simulink model "NominalEncounter"  (R2021b)
settings: Solver=ode45  StartTime=0.0  StopTime=90  RelTol=1e-3  EnableMultiTasking=on
undefined symbols (not defined in the file or in its folder): radarParamConverter, Subsystem
libraries: Tracked_Radar_Block x3, NominalTrajectory x2, BasicAircraftDynamicsBlock x2, GPS_INS_Block x2, CommonMetricsBlock x1, SLoWCBlock x1, WellClearMetricsBlock x1, StopConditionsBlock x1, aerolibutil x1, sph2cart x1
settings Model: Creator=JO20596  LastModifiedBy=lydiazeleke
settings SolverCC: AlgebraicLoopSolver=TrustRegion
settings DataIOCC: LimitDataPoints=on  MaxDataPoints=10000  SignalLoggingSaveFormat=ModelDataLogs  SaveState=on  ReturnWorkspaceOutputs=off  StateSaveName=xoutNew  OutputSaveName=youtNew
settings OptimizationCC: ExpressionDepthLimit=2147483647  LifeSpan=inf
settings DebuggingCC: UnderspecifiedInitializationDetection=Classic  MergeDetectMultiDrivingBlocksExec=none  SolverPrmCheckMsg=warning  FcnCallInpInsideContextMsg=warning  StateNameClashWarn=warning  SFUnexpectedBacktrackingDiag=warning  SFNoUnconditionalDefaultTransitionDiag=warning  SFExecutionAtInitializationDiag=none  SFMachineParentedDataDiag=warning  ArithmeticOperatorsInVariantConditions=warning
settings HardwareCC: ProdBitPerPointer=32  ProdBitPerSizeT=32  ProdBitPerPtrDiffT=32  ProdLargestAtomicFloat=None  ProdIntDivRoundTo=Undefined  ProdEndianess=Unspecified  ProdWordSize=32  ProdHWDeviceType=32-bit Generic
settings ModelReferenceCC: PropagateSignalLabelsOutOfModel=off
settings SFSimCC: SimUseLocalCustomCode=off  CustomCodeUndefinedFunction=UseInterfaceOnly
settings RTWCC: RTWUseLocalCustomCode=off
settings CodeAppCC: StateflowObjectComments=on
settings GRTTargetCC: TargetLangStandard=C89/C90 (ANSI)  CombineOutputUpdateFcns=off  GRTInterface=on
settings ConfigComp: CovMetricSettings=dw  CovSaveCumulativeToWorkspaceVar=on  CovSaveSingleToWorkspaceVar=on  CovExternalEMLEnable=off

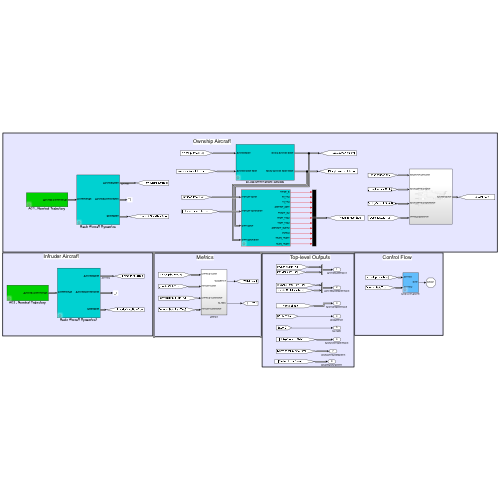
[thumbnail: Simulink's stored preview of the top-level diagram]
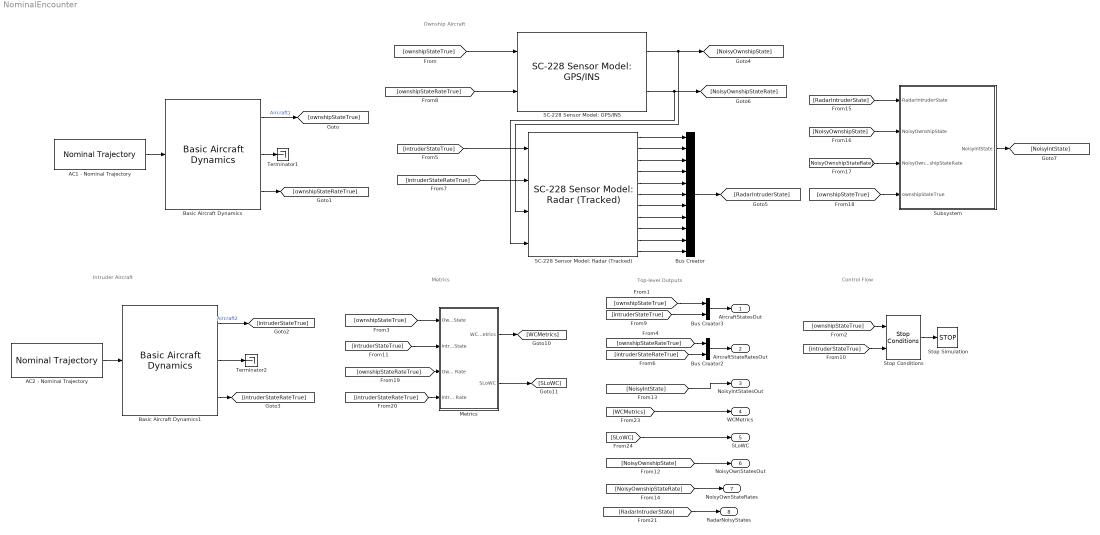
== system NominalEncounter ==
  note: Metrics
  note: Control Flow
  note: Top-level Outputs
  note: Ownship Aircraft
  note: Intruder Aircraft
  AC1 - Nominal Trajectory : NominalTrajectory/Nominal Trajectory  eventFilename=event1.mat  ts=.1
  AC2 - Nominal Trajectory : NominalTrajectory/Nominal Trajectory  eventFilename=event2.mat  ts=.1
  Basic Aircraft Dynamics : BasicAircraftDynamicsBlock/Basic Aircraft Dynamics  ts_dynamics=.1  v_ftps_0=ac1dyn_v_ftps  N_ft_0=ac1dyn_N_ft  E_ft_0=ac1dyn_E_ft  h_ft_0=ac1dyn_h_ft  psi_rad_0=ac1dyn_psi_rad  theta_rad_0=ac1dyn_theta_rad  phi_rad_0=ac1dyn_phi_rad  a_ftpss_0=ac1dyn_a_ftpss  v_ftps_max=ac1dyn_con.maxAirspeed_ftps  v_ftps_min=ac1dyn_con.minAirspeed_ftps  dv_ftpss_max=ac1dyn_con.maxAcceleration_ftpss  dv_ftpss_min=ac1dyn_con.minAcceleration_ftpss  dh_ftps_max=ac1dyn_con.maxVerticalRate_ftps  dh_ftps_min=ac1dyn_con.minVerticalRate_ftps  q_radps_max=ac1dyn_con.maxPitchRate_radps  phi_rad_max=ac1dyn_con.maxBankAngle_rad  dphi_radps_max=ac1dyn_con.maxRollRate_radps  r_radps_max=ac1dyn_con.maxYawRate_radps  pNUM=ac1dyn_con.dynamicsNumeratorRollRate  pDEN=ac1dyn_con.dynamicsDenominatorRollRate  hNUM=ac1dyn_con.dynamicsNumeratorVerticalRate  hDEN=ac1dyn_con.dynamicsDenominatorVerticalRate  rNUM=ac1dyn_con.dynamicsNumeratorYawRate  rDEN=ac1dyn_con.dynamicsDenominatorYawRate  lat0_rad=ac1dyn_lat0_rad  lon0_rad=ac1dyn_lon0_rad  alt_ft=ac1dyn_alt0_ft
  Basic Aircraft Dynamics1 : BasicAircraftDynamicsBlock/Basic Aircraft Dynamics  ts_dynamics=.1  v_ftps_0=ac2dyn_v_ftps  N_ft_0=ac2dyn_N_ft  E_ft_0=ac2dyn_E_ft  h_ft_0=ac2dyn_h_ft  psi_rad_0=ac2dyn_psi_rad  theta_rad_0=ac2dyn_theta_rad  phi_rad_0=ac2dyn_phi_rad  a_ftpss_0=ac2dyn_a_ftpss  v_ftps_max=ac2dyn_con.maxAirspeed_ftps  v_ftps_min=ac2dyn_con.minAirspeed_ftps  dv_ftpss_max=ac2dyn_con.maxAcceleration_ftpss  dv_ftpss_min=ac2dyn_con.minAcceleration_ftpss  dh_ftps_max=ac2dyn_con.maxVerticalRate_ftps  dh_ftps_min=ac2dyn_con.minVerticalRate_ftps  q_radps_max=ac2dyn_con.maxPitchRate_radps  phi_rad_max=ac2dyn_con.maxBankAngle_rad  dphi_radps_max=ac2dyn_con.maxRollRate_radps  r_radps_max=ac2dyn_con.maxYawRate_radps  pNUM=ac2dyn_con.dynamicsNumeratorRollRate  pDEN=ac2dyn_con.dynamicsDenominatorRollRate  hNUM=ac2dyn_con.dynamicsNumeratorVerticalRate  hDEN=ac2dyn_con.dynamicsDenominatorVerticalRate  rNUM=ac2dyn_con.dynamicsNumeratorYawRate  rDEN=ac2dyn_con.dynamicsDenominatorYawRate  lat0_rad=ac2dyn_lat0_rad  lon0_rad=ac2dyn_lon0_rad  alt_ft=ac2dyn_alt0_ft
  Bus Creator : BusCreator  Inputs=11
  Bus Creator2 : BusCreator  Inputs=2
  Bus Creator3 : BusCreator  Inputs=2
  Metrics : Subsystem
  SC-228 Sensor Model: GPS/INS : GPS_INS_Block/SC-228 Sensor Model: GPS//INS  dt_s=uas_own_dt_s  perfect=uas_own_usePerfectAlt  lat0_rad=ac1dyn_lat0_rad  lon0_rad=ac1dyn_lon0_rad  alt0_ft=ac1dyn_alt0_ft  vx_random_stddev_ftps=uas_own_vy_random_stddev_ftps  vx_bias_ftps=uas_own_vy_bias_ftps  vx_tau_s=uas_own_vy_tau_s  seed4=uas_own_seed4  vy_random_stddev_ftps=uas_own_vx_random_stddev_ftps  vy_bias_ftps=uas_own_vx_bias_ftps  vy_tau_s=uas_own_vx_tau_s  seed5=uas_own_seed5  psi_random_stddev_rad=uas_own_psi_random_stddev_rad  seed1=uas_own_seed1  phi_random_stddev_rad=uas_own_phi_random_stddev_rad  seed2=uas_own_seed2  theta_random_stddev_rad=uas_own_theta_random_stddev_rad  seed3=uas_own_seed3  seed6=uas_own_seed6  y_random_stddev_ft=uas_own_y_random_stddev_ft  y_bias_ft=uas_own_y_bias_ft  y_tau_s=uas_own_y_tau_s  seed7=uas_own_seed7  x_random_stddev_ft=uas_own_x_random_stddev_ft  x_bias_ft=uas_own_x_bias_ft  x_tau_s=uas_own_x_tau_s  seed8=uas_own_seed8  seed9=uas_own_seed9  seed10=uas_own_seed10  altQuant_ft=uas_own_altQuant_ft
  SC-228 Sensor Model: Radar (Tracked) : Tracked_Radar_Block/SC-228 Sensor Model: Radar (Tracked)  dt_s=uas_rdr_trckd_dt_s  lat0_rad=ac1dyn_lat0_rad  lon0_rad=ac1dyn_lon0_rad  alt0_ft=ac1dyn_alt0_ft  sns_for_azimuth_deg=uas_rdr_trckd_sns_for_azimuth_deg  sns_for_elevation_deg=uas_rdr_trckd_sns_for_elevation_deg  debugMode=uas_rdr_trckd_debugMode  rng_random_stddev_ft=uas_rdr_trckd_rng_random_stddev_ft  rng_bias_ft=uas_rdr_trckd_rng_bias_ft  rng_tau_s=uas_rdr_trckd_rng_tau_s  seed1=uas_rdr_trckd_seed1  RCPR_Mode=uas_rdr_trckd_RCPR_Mode  RCPR_Range_ft=uas_rdr_trckd_RCPR_Range_ft  az_random_stddev_rad=uas_rdr_trckd_az_random_stddev_rad  az_bias_rad=uas_rdr_trckd_az_bias_rad  az_tau_s=uas_rdr_trckd_az_tau_s  seed2=uas_rdr_trckd_seed2  el_random_stddev_rad=uas_rdr_trckd_el_random_stddev_rad  el_bias_rad=uas_rdr_trckd_el_bias_rad  el_tau_s=uas_rdr_trckd_el_tau_s  seed3=uas_rdr_trckd_seed3  rngdot_random_stddev_ftps=uas_rdr_trckd_rngdot_random_stddev_ftps  rngdot_bias_ftps=uas_rdr_trckd_rngdot_bias_ftps  rngdot_tau_s=uas_rdr_trckd_rngdot_tau_s  seed4=uas_rdr_trckd_seed4  covRAE=uas_rdr_trckd_reported_errorCovRAE
  Stop Conditions : StopConditionsBlock/Stop Conditions  range_limit_ft=stop_range_ft  altitude_limit_ft=stop_altitude_ft
  Stop Simulation : Stop
  Subsystem : Subsystem  AncestorBlock=radarParamConverter/Subsystem
  Terminator1 : Terminator
  Terminator2 : Terminator
  AircraftStatesOut : Outport  VectorParamsAs1DForOutWhenUnconnected=off
  AircraftStateRatesOut : Outport  Port=2  VectorParamsAs1DForOutWhenUnconnected=off
  NoisyIntStatesOut : Outport  Port=3  VectorParamsAs1DForOutWhenUnconnected=off
  WCMetrics : Outport  Port=4  VectorParamsAs1DForOutWhenUnconnected=off
  SLoWC : Outport  Port=5  VectorParamsAs1DForOutWhenUnconnected=off
  NoisyOwnStatesOut : Outport  Port=6  VectorParamsAs1DForOutWhenUnconnected=off
  NoisyOwnStateRates : Outport  Port=7  VectorParamsAs1DForOutWhenUnconnected=off
  RadarNoisyStates : Outport  Port=8  VectorParamsAs1DForOutWhenUnconnected=off
  wires:
  Bus Creator2/1 -> AircraftStateRatesOut/1
  Stop Conditions/1 -> Stop Simulation/1
  [ownshipStateTrue] -> Stop Conditions/1
  [ownshipStateRateTrue] -> Bus Creator2/1
  [intruderStateRateTrue] -> Bus Creator2/2
  [intruderStateTrue] -> Stop Conditions/2
  [ownshipStateTrue] -> Metrics/1(Ownship State)
  [intruderStateTrue] -> Metrics/2(Intruder State)
  [ownshipStateRateTrue] -> Metrics/3(Ownship State Rate)
  [intruderStateRateTrue] -> Metrics/4(Intruder State Rate)
  Metrics/1(WCMetrics) -> [WCMetrics]
  Metrics/2(SLoWC) -> [SLoWC]
  [WCMetrics] -> WCMetrics/1
  [SLoWC] -> SLoWC/1
  Basic Aircraft Dynamics1/3 -> [intruderStateRateTrue]
  Basic Aircraft Dynamics/2 -> Terminator1/1
  AC1 - Nominal Trajectory/1 -> Basic Aircraft Dynamics/1
  Basic Aircraft Dynamics1/1 -> [intruderStateTrue]  "Aircraft2"
  Basic Aircraft Dynamics1/2 -> Terminator2/1
  AC2 - Nominal Trajectory/1 -> Basic Aircraft Dynamics1/1
  Basic Aircraft Dynamics/1 -> [ownshipStateTrue]  "Aircraft1"
  Basic Aircraft Dynamics/3 -> [ownshipStateRateTrue]
  [intruderStateTrue] -> SC-228 Sensor Model: Radar (Tracked)/1
  [NoisyIntState] -> NoisyIntStatesOut/1
  [ownshipStateTrue] -> Bus Creator3/1
  [intruderStateTrue] -> Bus Creator3/2
  Bus Creator3/1 -> AircraftStatesOut/1
  SC-228 Sensor Model: GPS/INS/1 -> SC-228 Sensor Model: Radar (Tracked)/3, [NoisyOwnshipState]
  SC-228 Sensor Model: GPS/INS/2 -> SC-228 Sensor Model: Radar (Tracked)/4, [NoisyOwnshipStateRate]
  [ownshipStateTrue] -> SC-228 Sensor Model: GPS/INS/1
  [ownshipStateRateTrue] -> SC-228 Sensor Model: GPS/INS/2
  [intruderStateRateTrue] -> SC-228 Sensor Model: Radar (Tracked)/2
  [NoisyOwnshipStateRate] -> NoisyOwnStateRates/1
  [NoisyOwnshipState] -> NoisyOwnStatesOut/1
  SC-228 Sensor Model: Radar (Tracked)/1 -> Bus Creator/1
  SC-228 Sensor Model: Radar (Tracked)/2 -> Bus Creator/2
  SC-228 Sensor Model: Radar (Tracked)/3 -> Bus Creator/3
  SC-228 Sensor Model: Radar (Tracked)/4 -> Bus Creator/4
  SC-228 Sensor Model: Radar (Tracked)/5 -> Bus Creator/5
  SC-228 Sensor Model: Radar (Tracked)/6 -> Bus Creator/6
  SC-228 Sensor Model: Radar (Tracked)/7 -> Bus Creator/7
  SC-228 Sensor Model: Radar (Tracked)/8 -> Bus Creator/8
  SC-228 Sensor Model: Radar (Tracked)/9 -> Bus Creator/9
  SC-228 Sensor Model: Radar (Tracked)/10 -> Bus Creator/10
  SC-228 Sensor Model: Radar (Tracked)/11 -> Bus Creator/11
  Bus Creator/1 -> [RadarIntruderState]
  [RadarIntruderState] -> Subsystem/1(RadarIntruderState)
  [NoisyOwnshipState] -> Subsystem/2(NoisyOwnshipState)
  [NoisyOwnshipStateRate] -> Subsystem/3(NoisyOwnshipStateRate)
  Subsystem/1(NoisyIntState) -> [NoisyIntState]
  [ownshipStateTrue] -> Subsystem/4(ownshipStateTrue)
  [RadarIntruderState] -> RadarNoisyStates/1

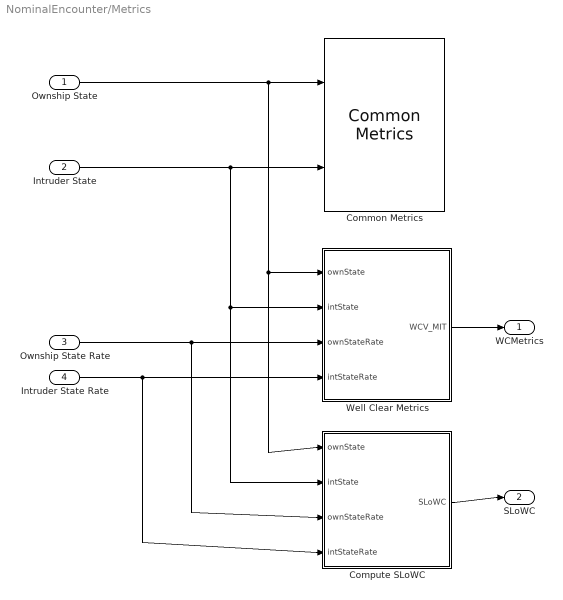
== system NominalEncounter/Metrics ==
  Ownship State : Inport
  Intruder State : Inport  Port=2
  Ownship State Rate : Inport  Port=3
  Intruder State Rate : Inport  Port=4
  Common Metrics : CommonMetricsBlock/Common Metrics
  Compute SLoWC : Subsystem  mask{DMOD=4000, tauMod=35, altDiff=450}
      mask prompts: altDiff "Altitude Difference Threshold:"
  Well Clear Metrics : Subsystem
  WCMetrics : Outport  VectorParamsAs1DForOutWhenUnconnected=off
  SLoWC : Outport  Port=2  VectorParamsAs1DForOutWhenUnconnected=off
  wires:
  Ownship State/1 -> Common Metrics/1, Well Clear Metrics/1(ownState), Compute SLoWC/1(ownState)
  Intruder State/1 -> Common Metrics/2, Well Clear Metrics/2(intState), Compute SLoWC/2(intState)
  Ownship State Rate/1 -> Well Clear Metrics/3(ownStateRate), Compute SLoWC/3(ownStateRate)
  Intruder State Rate/1 -> Well Clear Metrics/4(intStateRate), Compute SLoWC/4(intStateRate)
  Well Clear Metrics/1(WCV_MIT) -> WCMetrics/1
  Compute SLoWC/1(SLoWC) -> SLoWC/1

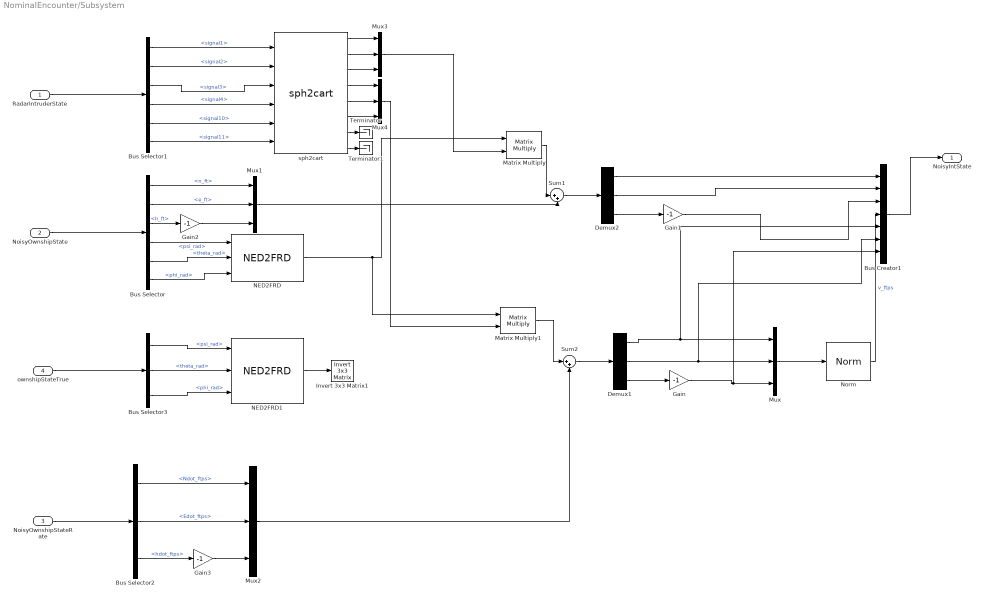
== system NominalEncounter/Subsystem ==
  RadarIntruderState : Inport
  NoisyOwnshipState : Inport  Port=2  OutDataTypeStr=Bus: AircraftState
  NoisyOwnshipStateRate : Inport  Port=3  OutDataTypeStr=Bus: AircraftStateRate
  ownshipStateTrue : Inport  Port=4  OutDataTypeStr=Bus: AircraftState
  Bus Creator1 : BusCreator  Inputs=7
  Bus Selector : BusSelector  OutputSignals=n_ft,e_ft,h_ft,psi_rad,theta_rad,phi_rad
  Bus Selector1 : BusSelector  OutputSignals=signal1,signal2,signal3,signal4,signal10,signal11
  Bus Selector2 : BusSelector  OutputSignals=Ndot_ftps,Edot_ftps,hdot_ftps
  Bus Selector3 : BusSelector  OutputSignals=psi_rad,theta_rad,phi_rad
  Demux1 : Demux  Outputs=3
  Demux2 : Demux  Outputs=3
  Gain{,1..3} (4 alike) : Gain  Gain=-1
  Invert 3x3 Matrix1 : aerolibutil/Invert  3x3 Matrix
  Matrix Multiply : Product  Multiplication=Matrix(*)
  Matrix Multiply1 : Product  Multiplication=Matrix(*)
  Mux{,1..4} (5 alike) : Mux  Inputs=3
  NED2FRD : Tracked_Radar_Block/SC-228 Sensor Model: Radar (Tracked)/NED2FRD  SystemSampleTime=-1  VariantActivationTime=update diagram  Latency=0  AutoFrameSizeCalculation=off
  NED2FRD1 : Tracked_Radar_Block/SC-228 Sensor Model: Radar (Tracked)/NED2FRD  SystemSampleTime=-1  VariantActivationTime=update diagram  Latency=0  AutoFrameSizeCalculation=off
  Norm : GPS_INS_Block/SC-228 Sensor Model: GPS//INS/Norm  SystemSampleTime=-1  VariantActivationTime=update diagram  Latency=0  AutoFrameSizeCalculation=off
  Sum1 : Sum  Inputs=|++
  Sum2 : Sum  Inputs=|++
  Terminator : Terminator
  Terminator1 : Terminator
  sph2cart : sph2cart/sph2cart  SystemSampleTime=-1  VariantActivationTime=update diagram  Latency=0  AutoFrameSizeCalculation=off
      settings: SourceProductName=CASSATTv6: Signals Library
  NoisyIntState : Outport  VectorParamsAs1DForOutWhenUnconnected=off
  wires:
  NoisyOwnshipState/1 -> Bus Selector/1
  RadarIntruderState/1 -> Bus Selector1/1
  NoisyOwnshipStateRate/1 -> Bus Selector2/1
  Bus Selector/4 -> NED2FRD/1  "<psi_rad>"
  Bus Selector/5 -> NED2FRD/2  "<theta_rad>"
  Bus Selector/6 -> NED2FRD/3  "<phi_rad>"
  Bus Selector/1 -> Mux1/1  "<n_ft>"
  Bus Selector/2 -> Mux1/2  "<e_ft>"
  Bus Selector2/1 -> Mux2/1  "<Ndot_ftps>"
  Bus Selector2/2 -> Mux2/2  "<Edot_ftps>"
  Matrix Multiply/1 -> Sum1/1
  Mux1/1 -> Sum1/2
  Sum1/1 -> Demux2/1
  Sum2/1 -> Demux1/1
  Mux2/1 -> Sum2/2
  Matrix Multiply1/1 -> Sum2/1
  Demux2/2 -> Bus Creator1/2
  Demux1/1 -> Bus Creator1/5, Mux/1
  Demux1/2 -> Bus Creator1/6, Mux/2
  Mux/1 -> Norm/1
  Demux1/3 -> Gain/1
  Demux2/3 -> Gain1/1
  Gain1/1 -> Bus Creator1/3
  Bus Selector1/1 -> sph2cart/1  "<signal1>"
  Bus Selector1/2 -> sph2cart/2  "<signal2>"
  sph2cart/1 -> Mux3/1
  Mux3/1 -> Matrix Multiply/2
  Mux4/1 -> Matrix Multiply1/2
  Demux2/1 -> Bus Creator1/1
  Bus Creator1/1 -> NoisyIntState/1
  Bus Selector1/3 -> sph2cart/3  "<signal3>"
  Bus Selector1/4 -> sph2cart/4  "<signal4>"
  Bus Selector1/5 -> sph2cart/5  "<signal10>"
  Bus Selector1/6 -> sph2cart/6  "<signal11>"
  sph2cart/2 -> Mux3/2
  sph2cart/3 -> Mux3/3
  sph2cart/4 -> Mux4/1
  sph2cart/5 -> Mux4/2
  sph2cart/6 -> Mux4/3
  sph2cart/7 -> Terminator/1
  sph2cart/8 -> Terminator1/1
  Gain/1 -> Bus Creator1/7, Mux/3
  Norm/1 -> Bus Creator1/4  "v_ftps"
  Bus Selector/3 -> Gain2/1  "<h_ft>"
  Gain2/1 -> Mux1/3
  Bus Selector2/3 -> Gain3/1  "<hdot_ftps>"
  Gain3/1 -> Mux2/3
  NED2FRD1/1 -> Invert 3x3 Matrix1/1
  Bus Selector3/1 -> NED2FRD1/1  "<psi_rad>"
  Bus Selector3/2 -> NED2FRD1/2  "<theta_rad>"
  Bus Selector3/3 -> NED2FRD1/3  "<phi_rad>"
  ownshipStateTrue/1 -> Bus Selector3/1
  NED2FRD/1 -> Matrix Multiply1/1, Matrix Multiply/1

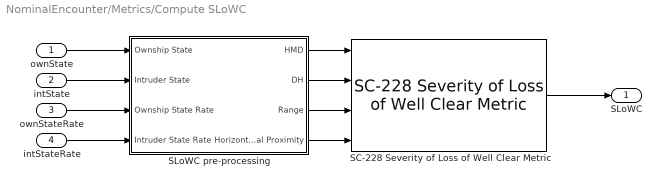
== system NominalEncounter/Metrics/Compute SLoWC ==
  ownState : Inport
  intState : Inport  Port=2
  ownStateRate : Inport  Port=3
  intStateRate : Inport  Port=4
  SC-228 Severity of Loss of Well Clear Metric : SLoWCBlock/SC-228 Severity of Loss of Well Clear Metric  DMOD=DMOD  altDiffThreshold=altDiff
  SLoWC pre-processing : Subsystem
  SLoWC : Outport  VectorParamsAs1DForOutWhenUnconnected=off
  wires:
  SLoWC pre-processing/2(DH) -> SC-228 Severity of Loss of Well Clear Metric/2
  SC-228 Severity of Loss of Well Clear Metric/1 -> SLoWC/1
  SLoWC pre-processing/1(HMD) -> SC-228 Severity of Loss of Well Clear Metric/1
  ownState/1 -> SLoWC pre-processing/1(Ownship State)
  SLoWC pre-processing/4(Horizontal Proximity) -> SC-228 Severity of Loss of Well Clear Metric/4
  SLoWC pre-processing/3(Range) -> SC-228 Severity of Loss of Well Clear Metric/3
  intState/1 -> SLoWC pre-processing/2(Intruder State)
  intStateRate/1 -> SLoWC pre-processing/4(Intruder State Rate)
  ownStateRate/1 -> SLoWC pre-processing/3(Ownship State Rate)

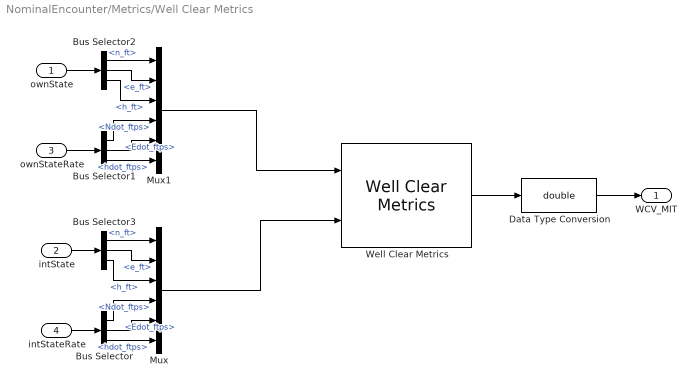
== system NominalEncounter/Metrics/Well Clear Metrics ==
  ownState : Inport  OutDataTypeStr=Bus: AircraftState
  intState : Inport  Port=2  OutDataTypeStr=Bus: AircraftState
  ownStateRate : Inport  Port=3  OutDataTypeStr=Bus: AircraftStateRate
  intStateRate : Inport  Port=4  OutDataTypeStr=Bus: AircraftStateRate
  Bus Selector : BusSelector  OutputSignals=Ndot_ftps,Edot_ftps,hdot_ftps
  Bus Selector1 : BusSelector  OutputSignals=Ndot_ftps,Edot_ftps,hdot_ftps
  Bus Selector2 : BusSelector  OutputSignals=n_ft,e_ft,h_ft
  Bus Selector3 : BusSelector  OutputSignals=n_ft,e_ft,h_ft
  Data Type Conversion : DataTypeConversion  OutDataTypeStr=double
  Mux : Mux  Inputs=6
  Mux1 : Mux  Inputs=6
  Well Clear Metrics : WellClearMetricsBlock/Well Clear Metrics  tauThreshold=wcm_modTau  hmdThreshold=wcm_HMD  tauVThreshold=wcm_TOCA  altThreshold=wcm_altThresh  rngThreshold=wcm_rangeThresh
  WCV_MIT : Outport  VectorParamsAs1DForOutWhenUnconnected=off
  wires:
  Well Clear Metrics/1 -> Data Type Conversion/1
  intStateRate/1 -> Bus Selector/1
  ownStateRate/1 -> Bus Selector1/1
  ownState/1 -> Bus Selector2/1
  intState/1 -> Bus Selector3/1
  Bus Selector3/1 -> Mux/1  "<n_ft>"
  Bus Selector3/2 -> Mux/2  "<e_ft>"
  Bus Selector3/3 -> Mux/3  "<h_ft>"
  Bus Selector/1 -> Mux/4  "<Ndot_ftps>"
  Bus Selector/2 -> Mux/5  "<Edot_ftps>"
  Bus Selector/3 -> Mux/6  "<hdot_ftps>"
  Bus Selector2/1 -> Mux1/1  "<n_ft>"
  Bus Selector2/2 -> Mux1/2  "<e_ft>"
  Bus Selector2/3 -> Mux1/3  "<h_ft>"
  Bus Selector1/3 -> Mux1/6  "<hdot_ftps>"
  Bus Selector1/1 -> Mux1/4  "<Ndot_ftps>"
  Bus Selector1/2 -> Mux1/5  "<Edot_ftps>"
  Mux1/1 -> Well Clear Metrics/1
  Mux/1 -> Well Clear Metrics/2
  Data Type Conversion/1 -> WCV_MIT/1

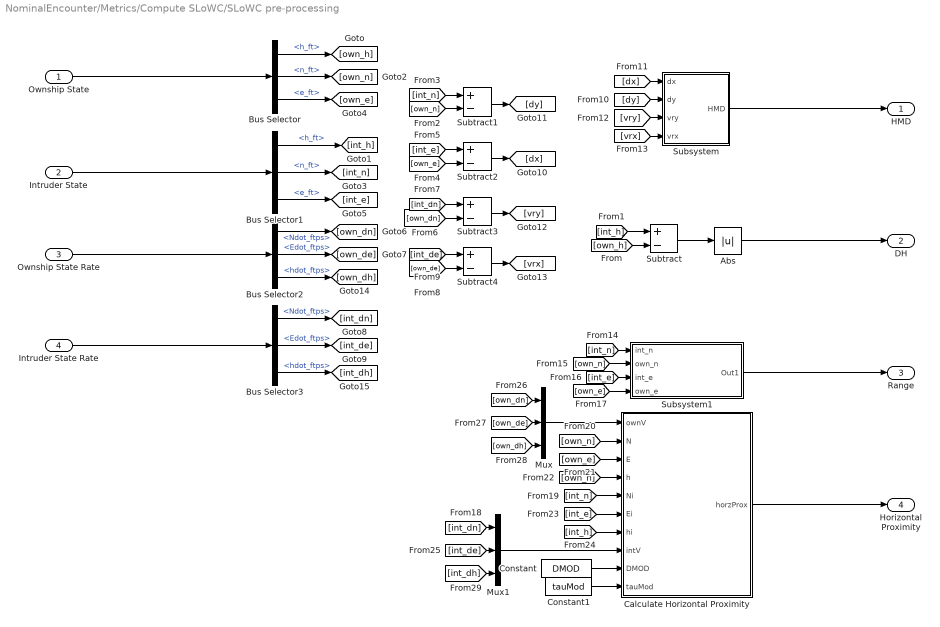
== system NominalEncounter/Metrics/Compute SLoWC/SLoWC pre-processing ==
  Ownship State : Inport
  Intruder State : Inport  Port=2
  Ownship State Rate : Inport  Port=3
  Intruder State Rate : Inport  Port=4
  Abs : Abs
  Bus Selector : BusSelector  OutputSignals=h_ft,n_ft,e_ft
  Bus Selector1 : BusSelector  OutputSignals=h_ft,n_ft,e_ft
  Bus Selector2 : BusSelector  OutputSignals=Ndot_ftps,Edot_ftps,hdot_ftps
  Bus Selector3 : BusSelector  OutputSignals=Ndot_ftps,Edot_ftps,hdot_ftps
  Calculate Horizontal Proximity : MATLAB Function  TreatAsAtomicUnit=on
  Constant : Constant  Value=DMOD
  Constant1 : Constant  Value=tauMod
  Mux : Mux  Inputs=3
  Mux1 : Mux  Inputs=3
  Subsystem : Subsystem
  Subsystem1 : Subsystem
  Subtract{,1..4} (5 alike) : Sum  Inputs=+-
  HMD : Outport  VectorParamsAs1DForOutWhenUnconnected=off
  DH : Outport  Port=2  VectorParamsAs1DForOutWhenUnconnected=off
  Range : Outport  Port=3  VectorParamsAs1DForOutWhenUnconnected=off
  Horizontal Proximity : Outport  Port=4  VectorParamsAs1DForOutWhenUnconnected=off
  wires:
  Subtract/1 -> Abs/1
  [own_dh] -> Mux/3
  Bus Selector/1 -> [own_h]  "<h_ft>"
  [own_dn] -> Subtract3/2
  Bus Selector1/3 -> [int_e]  "<e_ft>"
  [int_n] -> Calculate Horizontal Proximity/5(Ni)
  Bus Selector3/3 -> [int_dh]  "<hdot_ftps>"
  [int_h] -> Calculate Horizontal Proximity/7(hi)
  [int_e] -> Subtract2/1
  [own_h] -> Subtract/2
  Intruder State/1 -> Bus Selector1/1
  [own_n] -> Subtract1/2
  Constant/1 -> Calculate Horizontal Proximity/9(DMOD)
  [own_e] -> Subtract2/2
  [int_dh] -> Mux1/3
  Subtract4/1 -> [vrx]
  [int_h] -> Subtract/1
  Bus Selector1/1 -> [int_h]  "<h_ft>"
  [vry] -> Subsystem/3(vry)
  [own_n] -> Calculate Horizontal Proximity/2(N)
  Bus Selector3/1 -> [int_dn]  "<Ndot_ftps>"
  Subtract2/1 -> [dx]
  Bus Selector1/2 -> [int_n]  "<n_ft>"
  Bus Selector/2 -> [own_n]  "<n_ft>"
  Subtract3/1 -> [vry]
  [int_e] -> Subsystem1/3(int_e)
  [own_de] -> Mux/2
  Mux1/1 -> Calculate Horizontal Proximity/8(intV)
  Subtract1/1 -> [dy]
  [own_h] -> Calculate Horizontal Proximity/4(h)
  [dy] -> Subsystem/2(dy)
  [own_n] -> Subsystem1/2(own_n)
  [int_dn] -> Mux1/1
  Subsystem/1(HMD) -> HMD/1
  Bus Selector2/2 -> [own_de]  "<Edot_ftps>"
  [int_n] -> Subtract1/1
  Bus Selector2/3 -> [own_dh]  "<hdot_ftps>"
  [int_de] -> Subtract4/1
  Constant1/1 -> Calculate Horizontal Proximity/10(tauMod)
  Bus Selector/3 -> [own_e]  "<e_ft>"
  Subsystem1/1(Out1) -> Range/1
  [int_n] -> Subsystem1/1("int_n ")
  [int_e] -> Calculate Horizontal Proximity/6(Ei)
  [own_de] -> Subtract4/2
  Bus Selector3/2 -> [int_de]  "<Edot_ftps>"
  Mux/1 -> Calculate Horizontal Proximity/1(ownV)
  [dx] -> Subsystem/1("dx ")
  [int_dn] -> Subtract3/1
  Intruder State Rate/1 -> Bus Selector3/1
  [vrx] -> Subsystem/4(vrx)
  [own_dn] -> Mux/1
  Bus Selector2/1 -> [own_dn]  "<Ndot_ftps>"
  Abs/1 -> DH/1
  [own_e] -> Calculate Horizontal Proximity/3(E)
  Calculate Horizontal Proximity/1(horzProx) -> Horizontal Proximity/1
  Ownship State/1 -> Bus Selector/1
  [int_de] -> Mux1/2
  [own_e] -> Subsystem1/4(own_e)
  Ownship State Rate/1 -> Bus Selector2/1

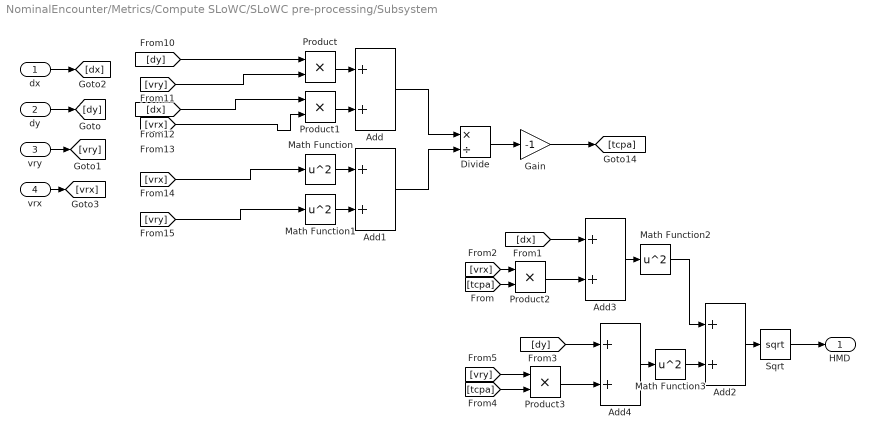
== system NominalEncounter/Metrics/Compute SLoWC/SLoWC pre-processing/Subsystem ==
  "dx " : Inport
  dy : Inport  Port=2
  vry : Inport  Port=3
  vrx : Inport  Port=4
  Add{,1..4} (5 alike) : Sum
  Divide : Product  Inputs=*/
  Gain : Gain  Gain=-1
  Math Function{,1..3} (4 alike) : Math  Operator=square  SignedPower=on  SaturateOnIntegerOverflow=on
  Product{,1..3} (4 alike) : Product
  Sqrt : Sqrt  SaturateOnIntegerOverflow=on
  HMD : Outport  VectorParamsAs1DForOutWhenUnconnected=off
  wires:
  Math Function1/1 -> Add1/2
  Gain/1 -> [tcpa]
  Add/1 -> Divide/1
  Math Function/1 -> Add1/1
  Product1/1 -> Add/2
  Product/1 -> Add/1
  [vrx] -> Math Function/1
  [vrx] -> Product1/2
  [dx] -> Product1/1
  Divide/1 -> Gain/1
  Add1/1 -> Divide/2
  [vry] -> Product/2
  [dy] -> Product/1
  [vry] -> Math Function1/1
  Sqrt/1 -> HMD/1
  Add2/1 -> Sqrt/1
  Math Function2/1 -> Add2/1
  Add3/1 -> Math Function2/1
  [dx] -> Add3/1
  [vrx] -> Product2/1
  Product2/1 -> Add3/2
  [tcpa] -> Product2/2
  Add4/1 -> Math Function3/1
  Math Function3/1 -> Add2/2
  Product3/1 -> Add4/2
  [dy] -> Add4/1
  [tcpa] -> Product3/2
  [vry] -> Product3/1
  "dx "/1 -> [dx]
  vrx/1 -> [vrx]
  vry/1 -> [vry]
  dy/1 -> [dy]

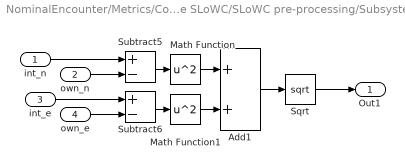
== system NominalEncounter/Metrics/Compute SLoWC/SLoWC pre-processing/Subsystem1 ==
  "int_n " : Inport
  own_n : Inport  Port=2
  int_e : Inport  Port=3
  own_e : Inport  Port=4
  Add1 : Sum
  Math Function : Math  Operator=square  SignedPower=on  SaturateOnIntegerOverflow=on
  Math Function1 : Math  Operator=square  SignedPower=on  SaturateOnIntegerOverflow=on
  Sqrt : Sqrt  SaturateOnIntegerOverflow=on
  Subtract5 : Sum  Inputs=+-
  Subtract6 : Sum  Inputs=+-
  Out1 : Outport  VectorParamsAs1DForOutWhenUnconnected=off
  wires:
  Math Function/1 -> Add1/1
  Add1/1 -> Sqrt/1
  Math Function1/1 -> Add1/2
  Subtract5/1 -> Math Function/1
  Sqrt/1 -> Out1/1
  Subtract6/1 -> Math Function1/1
  int_e/1 -> Subtract6/1
  own_n/1 -> Subtract5/2
  "int_n "/1 -> Subtract5/1
  own_e/1 -> Subtract6/2

== matlab function NominalEncounter/Metrics/Compute SLoWC/SLoWC pre-processing/Calculate Horizontal Proximity ==
  data: ownV input; N input; horzProx output; E input; h input; Ni input; Ei input; hi input; intV input; DMOD input; tauMod input
function horzProx = getHorzProx(ownV,N,E,h,Ni,Ei,hi,intV, DMOD, tauMod) 
% This block computes horizontal proximity (S_i in the Bihrle slide 3)

%Ri = [Ni-N; Ei-E; -(hi-h)];
Ri = [Ni-N; Ei-E; 0];

rangeRate = 0;

if(~isempty(Ri) && ~isempty(ownV) && ~isempty(intV))
    relVel = intV - ownV;
    rangeRate = dot(Ri/norm(Ri), relVel);
end

horzProx = max(DMOD, 0.5* (sqrt((rangeRate*tauMod)^2 + 4*DMOD^2) - rangeRate*tauMod) );
